simulink model "VelocityIntegratorBipolar"  (R2016a)
settings: Solver=VariableStepAuto  StartTime=0.0  StopTime=25  RelTol=1e-3
libraries: fl_lib x40, elec_lib x8, nesl_utility x4, pe_lib x2
settings Model: Creator=Peter  LastModifiedBy=Peter

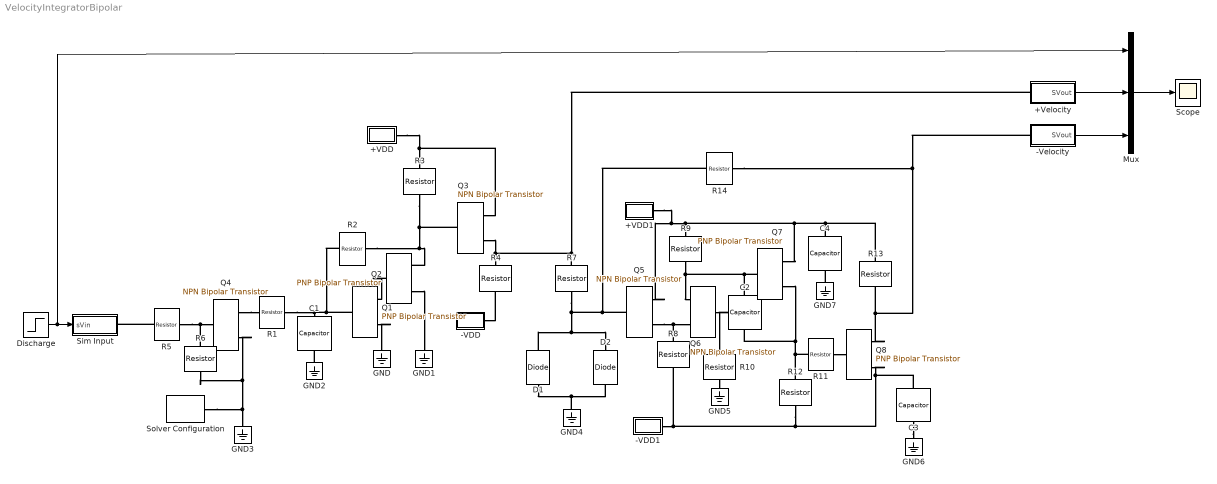
== system VelocityIntegratorBipolar ==
  +VDD : Subsystem
  +VDD1 : Subsystem
  +Velocity : Subsystem
  -VDD : Subsystem
  -VDD1 : Subsystem
  -Velocity : Subsystem
  C1 : fl_lib/Electrical/Electrical Elements/Capacitor  c=100e-6 F  r=1e-6 Ohm  g=0 1/Ohm  i_specify=off  i_priority=None  i=0 A  v_specify=off  v_priority=None  v=0 V  vc_specify=off  vc_priority=High  vc=0 V
  C2 : fl_lib/Electrical/Electrical Elements/Capacitor  c=560e-9 F  r=1e-6 Ohm  g=0 1/Ohm  i_specify=off  i_priority=None  i=0 A  v_specify=off  v_priority=None  v=0 V  vc_specify=off  vc_priority=High  vc=0 V
  C3 : fl_lib/Electrical/Electrical Elements/Capacitor  c=100e-9 F  r=1e-6 Ohm  g=0 1/Ohm  i_specify=off  i_priority=None  i=0 A  v_specify=off  v_priority=None  v=0 V  vc_specify=off  vc_priority=High  vc=0 V
  C4 : fl_lib/Electrical/Electrical Elements/Capacitor  c=100e-9 F  r=1e-6 Ohm  g=0 1/Ohm  i_specify=off  i_priority=None  i=0 A  v_specify=off  v_priority=None  v=0 V  vc_specify=off  vc_priority=High  vc=0 V
  D1 : pe_lib/Semiconductors/Fundamental Components/Diode  Vf=0.8 V  Ron=0.001 Ohm  Goff=1e-5 1/Ohm  N_series=1  N_parallel=1  Vf_equiv=0.8 V  Ron_equiv=0.001 Ohm  Goff_equiv=1e-5 1/Ohm
  D2 : pe_lib/Semiconductors/Fundamental Components/Diode  Vf=0.8 V  Ron=0.001 Ohm  Goff=1e-5 1/Ohm  N_series=1  N_parallel=1  Vf_equiv=0.8 V  Ron_equiv=0.001 Ohm  Goff_equiv=1e-5 1/Ohm
  Discharge : Step  Time=5  After=0  SampleTime=0
  GND{,1..7} (8 alike) : fl_lib/Electrical/Electrical Elements/Electrical Reference
  Mux : Mux  Inputs=3
  Q{1..2,7..8} (4 alike) : elec_lib/Semiconductor Devices/PNP Bipolar Transistor  parameterization=1  prmDatasheet=1  prmEquCoeff=1  BF=100  IS=1e-14 A  ec=1  VAF=200 V  hfe=100  hoe=5e-5 1/Ohm  Ic_h=-1 mA  Vce_h=-5 V  V1=-0.55 V  I1=-0.5 mA  BR=1  Tmeas=25 degC  RC=0.01 Ohm  RE=1e-4 Ohm  RB=1 Ohm  C_BC=5 pF  C_BE=5 pF  TF=0 us  TR=0 us  hfe_T2=125  XTB=0  V1_T2=-0.45 V  I1_T2=-0.5 mA  Tmeas2=125 degC  EG=1.11 eV  XTI=3  TdeviceDatasheet=25 degC  TdeviceEquCoeff=25 degC  Rth=[ 0 10 ] K/W  thermal_mass_parameterization=1  thermal_mass=[ 0 1 ] J/K  thermal_time_constant=[ 0 10 ] s  thermal_mass_initial_temperatures=[ 25 25 ] degC
  Q{3..6} (4 alike) : elec_lib/Semiconductor Devices/NPN Bipolar Transistor  parameterization=1  prmDatasheet=1  prmEquCoeff=1  BF=100  IS=1e-14 A  ec=1  VAF=200 V  hfe=100  hoe=5e-5 1/Ohm  Ic_h=1 mA  Vce_h=5 V  V1=0.55 V  I1=0.5 mA  BR=1  Tmeas=25 degC  RC=0.01 Ohm  RE=1e-4 Ohm  RB=1 Ohm  C_BC=5 pF  C_BE=5 pF  TF=0 us  TR=0 us  hfe_T2=125  XTB=0  V1_T2=0.45 V  I1_T2=0.5 mA  Tmeas2=125 degC  EG=1.11 eV  XTI=3  TdeviceDatasheet=25 degC  TdeviceEquCoeff=25 degC  Rth=[ 0 10 ] K/W  thermal_mass_parameterization=1  thermal_mass=[ 0 1 ] J/K  thermal_time_constant=[ 0 10 ] s  thermal_mass_initial_temperatures=[ 25 25 ] degC
  R1 : fl_lib/Electrical/Electrical Elements/Resistor  R=1 kOhm  i_specify=off  i_priority=None  i=0 A  v_specify=off  v_priority=None  v=0 V
  R10 : fl_lib/Electrical/Electrical Elements/Resistor  R=15 kOhm  i_specify=off  i_priority=None  i=0 A  v_specify=off  v_priority=None  v=0 V
  R11 : fl_lib/Electrical/Electrical Elements/Resistor  R=100 Ohm  i_specify=off  i_priority=None  i=0 A  v_specify=off  v_priority=None  v=0 V
  R{5,7,12,14} (4 alike) : fl_lib/Electrical/Electrical Elements/Resistor  R=30 kOhm  i_specify=off  i_priority=None  i=0 A  v_specify=off  v_priority=None  v=0 V
  R13 : fl_lib/Electrical/Electrical Elements/Resistor  R=3 kOhm  i_specify=off  i_priority=None  i=0 A  v_specify=off  v_priority=None  v=0 V
  R2 : fl_lib/Electrical/Electrical Elements/Resistor  R=220 kOhm  i_specify=off  i_priority=None  i=0 A  v_specify=off  v_priority=None  v=0 V
  R3 : fl_lib/Electrical/Electrical Elements/Resistor  R=10 kOhm  i_specify=off  i_priority=None  i=0 A  v_specify=off  v_priority=None  v=0 V
  R4 : fl_lib/Electrical/Electrical Elements/Resistor  R=20 kOhm  i_specify=off  i_priority=None  i=0 A  v_specify=off  v_priority=None  v=0 V
  R6 : fl_lib/Electrical/Electrical Elements/Resistor  R=100 kOhm  i_specify=off  i_priority=None  i=0 A  v_specify=off  v_priority=None  v=0 V
  R8 : fl_lib/Electrical/Electrical Elements/Resistor  R=100 kOhm  i_specify=off  i_priority=None  i=0 A  v_specify=off  v_priority=None  v=0 V
  R9 : fl_lib/Electrical/Electrical Elements/Resistor  R=10 kOhm  i_specify=off  i_priority=None  i=0 A  v_specify=off  v_priority=None  v=0 V
  Scope : Scope
  Sim Input : Subsystem
  Solver Configuration : nesl_utility/Solver Configuration  PhysicalDomain=network_engine_domain  SubClassName=solver  LeftPortType=input  RightPortType=generic  Accelerate=off  Tones=[]  Harmonics=[]  SimulateNoise=off  Profile=off  UseLocalSampling=off  EnableSwitchedLinearOptims=on  FrequencyDomain=off  UseCCode=off  RelTol=0.001  AbsTol=1e-06  MinStep=1e-09  ToWorkspace=off  RevertToSquareIcSolve=off  NumHomotopyIterations=100  PhasorMode=off  PhasorModeNumHarmonics=1  OverrideAbsTol=off  DoDC=off  ResidualTolerance=1e-09  UseLocalSolver=off  LocalSolverChoice=NE_BACKWARD_EULER_ADVANCER  LocalSolverSampleTime=0.001  DoFixedCost=off  MaxNonlinIter=3  MaxModeIter=2  LinearAlgebra=Sparse  DelaysMemoryBudget=1024  AutomaticFiltering=on  FilteringTimeConstant=0.001
  wires:
  Discharge/1 -> Mux/1, Sim Input/1(sVin)
  Mux/1 -> Scope/1
  +Velocity/1(SVout) -> Mux/2
  -Velocity/1(SVout) -> Mux/3
  connections:
  Q2/LConn1 -- Q1/RConn1
  Q1/RConn2 -- GND/LConn1
  Q2/RConn2 -- GND1/LConn1
  Q1/LConn1 -- R2/RConn1 -- R1/RConn1 -- C1/LConn1
  R3/RConn1 -- Q3/LConn1 -- Q2/RConn1 -- R2/LConn1
  +VDD/RConn1 -- Q3/RConn1 -- R3/LConn1
  Q3/RConn2 -- +Velocity/LConn1 -- R7/LConn1 -- R4/LConn1
  -VDD/RConn1 -- R4/RConn1
  Q4/RConn1 -- R1/LConn1
  Q4/RConn2 -- R6/RConn1 -- Solver Configuration/RConn1 -- GND3/LConn1
  GND2/LConn1 -- C1/RConn1
  R5/RConn1 -- R6/LConn1 -- Q4/LConn1
  R5/LConn1 -- Sim Input/RConn1
  D1/LConn1 -- GND4/LConn1 -- D2/RConn1
  D1/RConn1 -- R14/LConn1 -- Q5/LConn1 -- R7/RConn1 -- D2/LConn1
  Q5/RConn2 -- R8/LConn1 -- Q6/RConn2
  -VDD1/RConn1 -- C3/RConn1 -- Q8/RConn2 -- R12/RConn1 -- R8/RConn1
  R9/RConn1 -- C2/LConn1 -- Q7/LConn1 -- Q6/RConn1
  Q5/RConn1 -- +VDD1/RConn1 -- C4/LConn1 -- R13/LConn1 -- Q7/RConn1 -- R9/LConn1
  Q6/LConn1 -- R10/LConn1
  R10/RConn1 -- GND5/LConn1
  Q7/RConn2 -- R12/LConn1 -- R11/LConn1 -- C2/RConn1
  R11/RConn1 -- Q8/LConn1
  C3/LConn1 -- GND6/LConn1
  Q8/RConn1 -- -Velocity/LConn1 -- R14/RConn1 -- R13/RConn1
  GND7/LConn1 -- C4/RConn1

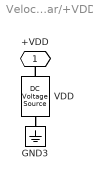
== system VelocityIntegratorBipolar/+VDD ==
  GND3 : fl_lib/Electrical/Electrical Elements/Electrical Reference
  VDD : fl_lib/Electrical/Electrical Sources/DC Voltage Source  v0=14.3 V
  +VDD : PMIOPort  Port=1  Side=Right
  connections:
  VDD/LConn1 -- +VDD/RConn1
  VDD/RConn1 -- GND3/LConn1

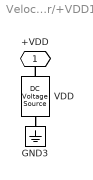
== system VelocityIntegratorBipolar/+VDD1 ==
  GND3 : fl_lib/Electrical/Electrical Elements/Electrical Reference
  VDD : fl_lib/Electrical/Electrical Sources/DC Voltage Source  v0=14.3 V
  +VDD : PMIOPort  Port=1  Side=Right
  connections:
  VDD/LConn1 -- +VDD/RConn1
  VDD/RConn1 -- GND3/LConn1

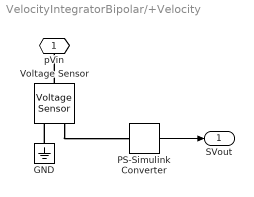
== system VelocityIntegratorBipolar/+Velocity ==
  GND : fl_lib/Electrical/Electrical Elements/Electrical Reference
  PS-Simulink Converter : nesl_utility/PS-Simulink Converter  PhysicalDomain=network_engine_domain  SubClassName=ps_output  LeftPortType=input  RightPortType=output  PseudoPeriodic=off  Frequencies=[]  Unit=V  AffineConversion=off
  Voltage Sensor : fl_lib/Electrical/Electrical Sensors/Voltage Sensor
  pVin : PMIOPort  Port=1  Side=Left
  SVout : Outport
  wires:
  PS-Simulink Converter/1 -> SVout/1
  connections:
  GND/LConn1 -- Voltage Sensor/RConn2
  Voltage Sensor/LConn1 -- pVin/RConn1
  Voltage Sensor/RConn1 -- PS-Simulink Converter/LConn1

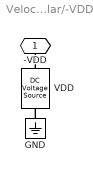
== system VelocityIntegratorBipolar/-VDD ==
  GND : fl_lib/Electrical/Electrical Elements/Electrical Reference
  VDD : fl_lib/Electrical/Electrical Sources/DC Voltage Source  v0=14.3 V
  -VDD : PMIOPort  Port=1  Side=Right
  connections:
  VDD/RConn1 -- -VDD/RConn1
  GND/LConn1 -- VDD/LConn1

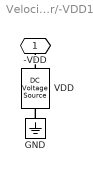
== system VelocityIntegratorBipolar/-VDD1 ==
  GND : fl_lib/Electrical/Electrical Elements/Electrical Reference
  VDD : fl_lib/Electrical/Electrical Sources/DC Voltage Source  v0=14.3 V
  -VDD : PMIOPort  Port=1  Side=Right
  connections:
  VDD/RConn1 -- -VDD/RConn1
  GND/LConn1 -- VDD/LConn1

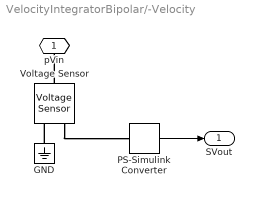
== system VelocityIntegratorBipolar/-Velocity ==
  GND : fl_lib/Electrical/Electrical Elements/Electrical Reference
  PS-Simulink Converter : nesl_utility/PS-Simulink Converter  PhysicalDomain=network_engine_domain  SubClassName=ps_output  LeftPortType=input  RightPortType=output  PseudoPeriodic=off  Frequencies=[]  Unit=V  AffineConversion=off
  Voltage Sensor : fl_lib/Electrical/Electrical Sensors/Voltage Sensor
  pVin : PMIOPort  Port=1  Side=Left
  SVout : Outport
  wires:
  PS-Simulink Converter/1 -> SVout/1
  connections:
  GND/LConn1 -- Voltage Sensor/RConn2
  Voltage Sensor/LConn1 -- pVin/RConn1
  Voltage Sensor/RConn1 -- PS-Simulink Converter/LConn1

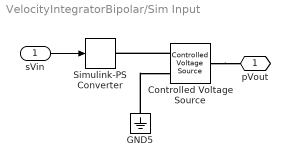
== system VelocityIntegratorBipolar/Sim Input ==
  sVin : Inport
  Controlled Voltage Source : fl_lib/Electrical/Electrical Sources/Controlled Voltage Source
  GND5 : fl_lib/Electrical/Electrical Elements/Electrical Reference
  Simulink-PS Converter : nesl_utility/Simulink-PS Converter  PhysicalDomain=network_engine_domain  SubClassName=ps_input  LeftPortType=input  RightPortType=output  PseudoPeriodic=off  Frequencies=[]  NoiseDistribution=none  NoiseParameters=[]  Unit=V  AffineConversion=off  InputFiltering=off  SimscapeFilterOrder=1  InputFilterTimeConstant=0.001  UdotUserProvided=1
  pVout : PMIOPort  Port=1  Side=Right
  wires:
  sVin/1 -> Simulink-PS Converter/1
  connections:
  Controlled Voltage Source/RConn1 -- Simulink-PS Converter/RConn1
  GND5/LConn1 -- Controlled Voltage Source/RConn2
  Controlled Voltage Source/LConn1 -- pVout/RConn1
